simulink model "Subsystem"  (R2021a)
settings: Solver=VariableStepAuto  StartTime=0.0  StopTime=10.0  RelTol=1e-3
settings Model: Creator=Nida  LastModifiedBy=Nida
settings DataIOCC: SaveOutput=off  SaveTime=off

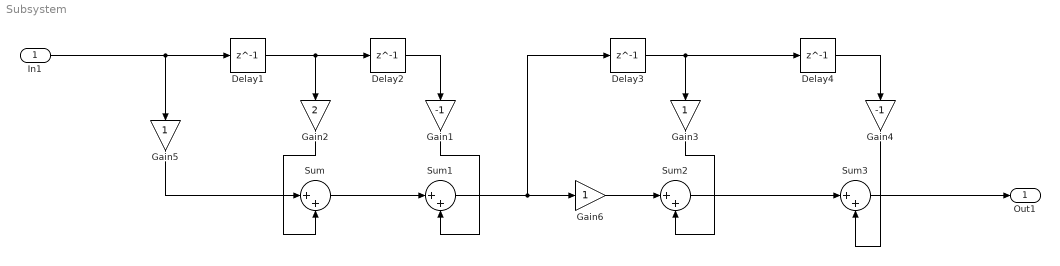
== system Subsystem ==
  In1 : Inport  OutDataTypeStr=double  PortDimensions=1  SampleTime=[0,1]
  Delay{1..4} (4 alike) : Delay  DelayLength=1
  Gain1 : Gain  Gain=-1
  Gain2 : Gain  Gain=2
  Gain3 : Gain
  Gain4 : Gain  Gain=-1
  Gain5 : Gain
  Gain6 : Gain
  Sum{,1..3} (4 alike) : Sum  Inputs=|++
  Out1 : Outport  OutDataTypeStr=double  PortDimensions=1  SampleTime=[0,1]
  wires:
  Sum2/1 -> Sum3/1
  Gain5/1 -> Sum/1
  Gain3/1 -> Sum2/2
  Delay4/1 -> Gain4/1
  Sum3/1 -> Out1/1
  In1/1 -> Gain5/1, Delay1/1
  Gain6/1 -> Sum2/1
  Delay3/1 -> Gain3/1, Delay4/1
  Sum1/1 -> Gain6/1, Delay3/1
  Gain2/1 -> Sum/2
  Delay2/1 -> Gain1/1
  Sum/1 -> Sum1/1
  Gain1/1 -> Sum1/2
  Delay1/1 -> Gain2/1, Delay2/1
  Gain4/1 -> Sum3/2
